simulink model "AAQuadModel"  (R2019b)
settings: Solver=VariableStepAuto  StartTime=0.0  StopTime=30.0  RelTol=1e-3
libraries: aerolibconvert2 x6, simulink x5, dspsigops x3, shared6dof x1, aerolibanim x1
settings Model: Creator=Antho  LastModifiedBy=Antho
settings SFSimCC: CustomCodeUndefinedFunction=UseInterfaceOnly

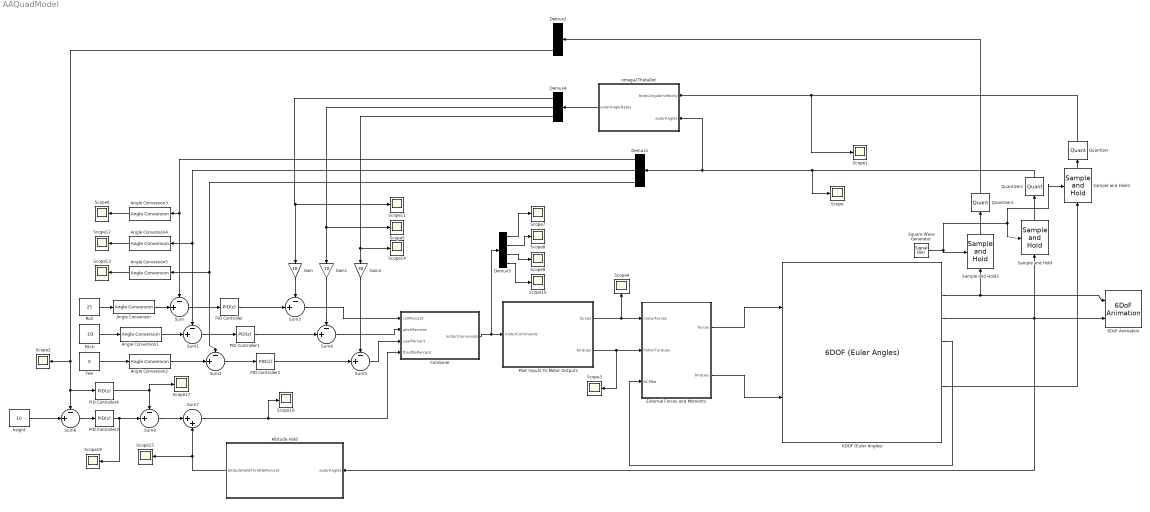
== system AAQuadModel ==
  6DOF (Euler Angles) : shared6dof/6DOF (Euler Angles)  units=Metric (MKS)  mtype=Fixed  rep=Euler Angles  xme_0=[0 0 0]  Vm_0=[0 0 0]  eul_0=[0 0 0]  pm_0=[0 0 0]  mass_0=0.5  mass_e=0.5  mass_f=2.0  inertia=[0.1 0 0; 0 0.1 0; 0 0 0.2]  inertia_e=eye(3)  inertia_f=2*eye(3)  k_quat=1.0  vre_flag=on  abi_flag=off  aMode=0  xme_statename=''  Vm_statename=''  eul_statename=''  quat_statename=''  pm_statename=''  mass_statename=''
      settings: SourceProductBaseCode=AE
  6DoF Animation : aerolibanim/6DoF Animation  u1=[0 4000 -2000 2000 -5000 -3000]  u2=0.1  u3=1.0  u4=[4000 0 -5000]  u5=Fixed position  u6=[2000 500 -3150]  u7=10  u8=on
      settings: SourceProductName=Aerospace Blockset
  Altitude Hold : MATLAB Function  TreatAsAtomicUnit=on
  Angle Conversion : aerolibconvert2/Angle Conversion  IU=deg  OU=rad
  Angle Conversion1 : aerolibconvert2/Angle Conversion  IU=deg  OU=rad
  Angle Conversion2 : aerolibconvert2/Angle Conversion  IU=deg  OU=rad
  Angle Conversion3 : aerolibconvert2/Angle Conversion  IU=rad  OU=deg
  Angle Conversion4 : aerolibconvert2/Angle Conversion  IU=rad  OU=deg
  Angle Conversion5 : aerolibconvert2/Angle Conversion  IU=rad  OU=deg
  "Combiner " : MATLAB Function  TreatAsAtomicUnit=on
  Demux1 : Demux  Outputs=3
  Demux2 : Demux  Outputs=3
  Demux3 : Demux
  Demux4 : Demux  Outputs=3
  "External Forces and Moments " : MATLAB Function  TreatAsAtomicUnit=on
  Gain : Gain  Gain=10
  Gain1 : Gain  Gain=10
  Gain2 : Gain  Gain=30
  PID Controller : simulink/Continuous/PID Controller  Controller=PID  Form=Parallel  TimeDomain=Discrete-time  SampleTime=0.02  IntegratorMethod=Forward Euler  FilterMethod=Forward Euler  ControllerParametersSource=internal  P=30  I=0.2  D=0  UseFilter=on  N=100  TunerSelectOption=Transfer Function Based (PID Tuner App)  InitialConditionSource=internal  InitialConditionForIntegrator=0  InitialConditionForFilter=0  DifferentiatorICPrevScaledInput=0  ExternalReset=none  TrackingMode=off  Kt=1  LimitOutput=on  UpperSaturationLimit=20  LowerSaturationLimit=-20  LinearizeAsGain=on  AntiWindupMode=none  Kb=1  POutMin=[]  POutMax=[]  IOutMin=[]  IOutMax=[]  DOutMin=[]  DOutMax=[]  NOutMin=[]  NOutMax=[]  SumOutMin=[]  SumOutMax=[]  SaturationOutMin=[]  SaturationOutMax=[]  PParamMin=[]  PParamMax=[]  IParamMin=[]  IParamMax=[]  DParamMin=[]  DParamMax=[]  NParamMin=[]  NParamMax=[]  KbParamMin=[]  KbParamMax=[]  KtParamMin=[]  KtParamMax=[]  KbOutMin=[]  KbOutMax=[]  KtOutMin=[]  KtOutMax=[]  IntegratorOutMin=[]  IntegratorOutMax=[]  FilterOutMin=[]  FilterOutMax=[]  SumI1OutMin=[]  SumI1OutMax=[]  SumI2OutMin=[]  SumI2OutMax=[]  SumI3OutMin=[]  SumI3OutMax=[]  SumI4OutMin=[]  SumI4OutMax=[]  SumDOutMin=[]  SumDOutMax=[]  DifferentiatorOutMin=[]  DifferentiatorOutMax=[]  FilterDiffOutCoefMin=[]  FilterDiffOutCoefMax=[]  ReciprocalOutMin=[]  ReciprocalOutMax=[]  SumDenOutMin=[]  SumDenOutMax=[]  SumNumOutMin=[]  SumNumOutMax=[]  DivideOutMin=[]  DivideOutMax=[]  IntegratorContinuousStateAttributes=''  IntegratorStateMustResolveToSignalObject=off  IntegratorRTWStateStorageClass=Auto  FilterContinuousStateAttributes=''  FilterStateMustResolveToSignalObject=off  FilterRTWStateStorageClass=Auto  ParallelPVariant=InternalParameters  IdealPVariant=Disabled  IVariant=InternalParameters  DVariant=InternalParameters  IntegratorVariant=Discrete  SatVariant=Enabled  AWVariant=Passthrough  PCopyVariant=Disabled  TRVariant=Disabled  FdbkBlocksVariant=Forward  IdealPFdbkVariant=Disabled  SatFdbkVariant=Disabled  DerivativeFilterVariant=ForwardEulerFilter  NVariant=InternalParameters  NCopyVariant=Disabled  FilterICVariant=InternalICsFilter  IntegratorICVariant=InternalICs  ExternalResetVariant=Disabled  TRSumVariant=Passthrough  SumFdbkVariant=Disabled  SumVariant=Sum_PID
  PID Controller1 : simulink/Continuous/PID Controller  Controller=PID  Form=Parallel  TimeDomain=Discrete-time  SampleTime=0.02  IntegratorMethod=Forward Euler  FilterMethod=Forward Euler  ControllerParametersSource=internal  P=30  I=0.2  D=0  UseFilter=on  N=100  TunerSelectOption=Transfer Function Based (PID Tuner App)  InitialConditionSource=internal  InitialConditionForIntegrator=0  InitialConditionForFilter=0  DifferentiatorICPrevScaledInput=0  ExternalReset=none  TrackingMode=off  Kt=1  LimitOutput=on  UpperSaturationLimit=20  LowerSaturationLimit=-20  LinearizeAsGain=on  AntiWindupMode=none  Kb=1  POutMin=[]  POutMax=[]  IOutMin=[]  IOutMax=[]  DOutMin=[]  DOutMax=[]  NOutMin=[]  NOutMax=[]  SumOutMin=[]  SumOutMax=[]  SaturationOutMin=[]  SaturationOutMax=[]  PParamMin=[]  PParamMax=[]  IParamMin=[]  IParamMax=[]  DParamMin=[]  DParamMax=[]  NParamMin=[]  NParamMax=[]  KbParamMin=[]  KbParamMax=[]  KtParamMin=[]  KtParamMax=[]  KbOutMin=[]  KbOutMax=[]  KtOutMin=[]  KtOutMax=[]  IntegratorOutMin=[]  IntegratorOutMax=[]  FilterOutMin=[]  FilterOutMax=[]  SumI1OutMin=[]  SumI1OutMax=[]  SumI2OutMin=[]  SumI2OutMax=[]  SumI3OutMin=[]  SumI3OutMax=[]  SumI4OutMin=[]  SumI4OutMax=[]  SumDOutMin=[]  SumDOutMax=[]  DifferentiatorOutMin=[]  DifferentiatorOutMax=[]  FilterDiffOutCoefMin=[]  FilterDiffOutCoefMax=[]  ReciprocalOutMin=[]  ReciprocalOutMax=[]  SumDenOutMin=[]  SumDenOutMax=[]  SumNumOutMin=[]  SumNumOutMax=[]  DivideOutMin=[]  DivideOutMax=[]  IntegratorContinuousStateAttributes=''  IntegratorStateMustResolveToSignalObject=off  IntegratorRTWStateStorageClass=Auto  FilterContinuousStateAttributes=''  FilterStateMustResolveToSignalObject=off  FilterRTWStateStorageClass=Auto  ParallelPVariant=InternalParameters  IdealPVariant=Disabled  IVariant=InternalParameters  DVariant=InternalParameters  IntegratorVariant=Discrete  SatVariant=Enabled  AWVariant=Passthrough  PCopyVariant=Disabled  TRVariant=Disabled  FdbkBlocksVariant=Forward  IdealPFdbkVariant=Disabled  SatFdbkVariant=Disabled  DerivativeFilterVariant=ForwardEulerFilter  NVariant=InternalParameters  NCopyVariant=Disabled  FilterICVariant=InternalICsFilter  IntegratorICVariant=InternalICs  ExternalResetVariant=Disabled  TRSumVariant=Passthrough  SumFdbkVariant=Disabled  SumVariant=Sum_PID
  PID Controller2 : simulink/Continuous/PID Controller  Controller=PID  Form=Parallel  TimeDomain=Discrete-time  SampleTime=0.02  IntegratorMethod=Forward Euler  FilterMethod=Forward Euler  ControllerParametersSource=internal  P=20  I=0.2  D=0  UseFilter=on  N=100  TunerSelectOption=Transfer Function Based (PID Tuner App)  InitialConditionSource=internal  InitialConditionForIntegrator=0  InitialConditionForFilter=0  DifferentiatorICPrevScaledInput=0  ExternalReset=none  TrackingMode=off  Kt=1  LimitOutput=on  UpperSaturationLimit=20  LowerSaturationLimit=-20  LinearizeAsGain=on  AntiWindupMode=none  Kb=1  POutMin=[]  POutMax=[]  IOutMin=[]  IOutMax=[]  DOutMin=[]  DOutMax=[]  NOutMin=[]  NOutMax=[]  SumOutMin=[]  SumOutMax=[]  SaturationOutMin=[]  SaturationOutMax=[]  PParamMin=[]  PParamMax=[]  IParamMin=[]  IParamMax=[]  DParamMin=[]  DParamMax=[]  NParamMin=[]  NParamMax=[]  KbParamMin=[]  KbParamMax=[]  KtParamMin=[]  KtParamMax=[]  KbOutMin=[]  KbOutMax=[]  KtOutMin=[]  KtOutMax=[]  IntegratorOutMin=[]  IntegratorOutMax=[]  FilterOutMin=[]  FilterOutMax=[]  SumI1OutMin=[]  SumI1OutMax=[]  SumI2OutMin=[]  SumI2OutMax=[]  SumI3OutMin=[]  SumI3OutMax=[]  SumI4OutMin=[]  SumI4OutMax=[]  SumDOutMin=[]  SumDOutMax=[]  DifferentiatorOutMin=[]  DifferentiatorOutMax=[]  FilterDiffOutCoefMin=[]  FilterDiffOutCoefMax=[]  ReciprocalOutMin=[]  ReciprocalOutMax=[]  SumDenOutMin=[]  SumDenOutMax=[]  SumNumOutMin=[]  SumNumOutMax=[]  DivideOutMin=[]  DivideOutMax=[]  IntegratorContinuousStateAttributes=''  IntegratorStateMustResolveToSignalObject=off  IntegratorRTWStateStorageClass=Auto  FilterContinuousStateAttributes=''  FilterStateMustResolveToSignalObject=off  FilterRTWStateStorageClass=Auto  ParallelPVariant=InternalParameters  IdealPVariant=Disabled  IVariant=InternalParameters  DVariant=InternalParameters  IntegratorVariant=Discrete  SatVariant=Enabled  AWVariant=Passthrough  PCopyVariant=Disabled  TRVariant=Disabled  FdbkBlocksVariant=Forward  IdealPFdbkVariant=Disabled  SatFdbkVariant=Disabled  DerivativeFilterVariant=ForwardEulerFilter  NVariant=InternalParameters  NCopyVariant=Disabled  FilterICVariant=InternalICsFilter  IntegratorICVariant=InternalICs  ExternalResetVariant=Disabled  TRSumVariant=Passthrough  SumFdbkVariant=Disabled  SumVariant=Sum_PID
  PID Controller3 : simulink/Continuous/PID Controller  Controller=PID  Form=Parallel  TimeDomain=Discrete-time  SampleTime=0.02  IntegratorMethod=Forward Euler  FilterMethod=Forward Euler  ControllerParametersSource=internal  P=3  I=1  D=0  UseFilter=on  N=100  TunerSelectOption=Transfer Function Based (PID Tuner App)  InitialConditionSource=internal  InitialConditionForIntegrator=0  InitialConditionForFilter=0  DifferentiatorICPrevScaledInput=0  ExternalReset=none  TrackingMode=off  Kt=1  LimitOutput=on  UpperSaturationLimit=20  LowerSaturationLimit=-20  LinearizeAsGain=on  AntiWindupMode=none  Kb=1  POutMin=[]  POutMax=[]  IOutMin=[]  IOutMax=[]  DOutMin=[]  DOutMax=[]  NOutMin=[]  NOutMax=[]  SumOutMin=[]  SumOutMax=[]  SaturationOutMin=[]  SaturationOutMax=[]  PParamMin=[]  PParamMax=[]  IParamMin=[]  IParamMax=[]  DParamMin=[]  DParamMax=[]  NParamMin=[]  NParamMax=[]  KbParamMin=[]  KbParamMax=[]  KtParamMin=[]  KtParamMax=[]  KbOutMin=[]  KbOutMax=[]  KtOutMin=[]  KtOutMax=[]  IntegratorOutMin=[]  IntegratorOutMax=[]  FilterOutMin=[]  FilterOutMax=[]  SumI1OutMin=[]  SumI1OutMax=[]  SumI2OutMin=[]  SumI2OutMax=[]  SumI3OutMin=[]  SumI3OutMax=[]  SumI4OutMin=[]  SumI4OutMax=[]  SumDOutMin=[]  SumDOutMax=[]  DifferentiatorOutMin=[]  DifferentiatorOutMax=[]  FilterDiffOutCoefMin=[]  FilterDiffOutCoefMax=[]  ReciprocalOutMin=[]  ReciprocalOutMax=[]  SumDenOutMin=[]  SumDenOutMax=[]  SumNumOutMin=[]  SumNumOutMax=[]  DivideOutMin=[]  DivideOutMax=[]  IntegratorContinuousStateAttributes=''  IntegratorStateMustResolveToSignalObject=off  IntegratorRTWStateStorageClass=Auto  FilterContinuousStateAttributes=''  FilterStateMustResolveToSignalObject=off  FilterRTWStateStorageClass=Auto  ParallelPVariant=InternalParameters  IdealPVariant=Disabled  IVariant=InternalParameters  DVariant=InternalParameters  IntegratorVariant=Discrete  SatVariant=Enabled  AWVariant=Passthrough  PCopyVariant=Disabled  TRVariant=Disabled  FdbkBlocksVariant=Forward  IdealPFdbkVariant=Disabled  SatFdbkVariant=Disabled  DerivativeFilterVariant=ForwardEulerFilter  NVariant=InternalParameters  NCopyVariant=Disabled  FilterICVariant=InternalICsFilter  IntegratorICVariant=InternalICs  ExternalResetVariant=Disabled  TRSumVariant=Passthrough  SumFdbkVariant=Disabled  SumVariant=Sum_PID
  PID Controller4 : simulink/Continuous/PID Controller  Controller=PID  Form=Parallel  TimeDomain=Discrete-time  SampleTime=0.02  IntegratorMethod=Forward Euler  FilterMethod=Forward Euler  ControllerParametersSource=internal  P=0  I=0  D=3  UseFilter=on  N=100  TunerSelectOption=Transfer Function Based (PID Tuner App)  InitialConditionSource=internal  InitialConditionForIntegrator=0  InitialConditionForFilter=0  DifferentiatorICPrevScaledInput=0  ExternalReset=none  TrackingMode=off  Kt=1  LimitOutput=on  UpperSaturationLimit=20  LowerSaturationLimit=-20  LinearizeAsGain=on  AntiWindupMode=none  Kb=1  POutMin=[]  POutMax=[]  IOutMin=[]  IOutMax=[]  DOutMin=[]  DOutMax=[]  NOutMin=[]  NOutMax=[]  SumOutMin=[]  SumOutMax=[]  SaturationOutMin=[]  SaturationOutMax=[]  PParamMin=[]  PParamMax=[]  IParamMin=[]  IParamMax=[]  DParamMin=[]  DParamMax=[]  NParamMin=[]  NParamMax=[]  KbParamMin=[]  KbParamMax=[]  KtParamMin=[]  KtParamMax=[]  KbOutMin=[]  KbOutMax=[]  KtOutMin=[]  KtOutMax=[]  IntegratorOutMin=[]  IntegratorOutMax=[]  FilterOutMin=[]  FilterOutMax=[]  SumI1OutMin=[]  SumI1OutMax=[]  SumI2OutMin=[]  SumI2OutMax=[]  SumI3OutMin=[]  SumI3OutMax=[]  SumI4OutMin=[]  SumI4OutMax=[]  SumDOutMin=[]  SumDOutMax=[]  DifferentiatorOutMin=[]  DifferentiatorOutMax=[]  FilterDiffOutCoefMin=[]  FilterDiffOutCoefMax=[]  ReciprocalOutMin=[]  ReciprocalOutMax=[]  SumDenOutMin=[]  SumDenOutMax=[]  SumNumOutMin=[]  SumNumOutMax=[]  DivideOutMin=[]  DivideOutMax=[]  IntegratorContinuousStateAttributes=''  IntegratorStateMustResolveToSignalObject=off  IntegratorRTWStateStorageClass=Auto  FilterContinuousStateAttributes=''  FilterStateMustResolveToSignalObject=off  FilterRTWStateStorageClass=Auto  ParallelPVariant=InternalParameters  IdealPVariant=Disabled  IVariant=InternalParameters  DVariant=InternalParameters  IntegratorVariant=Discrete  SatVariant=Enabled  AWVariant=Passthrough  PCopyVariant=Disabled  TRVariant=Disabled  FdbkBlocksVariant=Forward  IdealPFdbkVariant=Disabled  SatFdbkVariant=Disabled  DerivativeFilterVariant=ForwardEulerFilter  NVariant=InternalParameters  NCopyVariant=Disabled  FilterICVariant=InternalICsFilter  IntegratorICVariant=InternalICs  ExternalResetVariant=Disabled  TRSumVariant=Passthrough  SumFdbkVariant=Disabled  SumVariant=Sum_PID
  Pilot Inputs To Motor Outputs : MATLAB Function  TreatAsAtomicUnit=on
  Pitch : Constant  Value=-10
  Quantizer : Quantizer  QuantizationInterval=0.00003  LinearizeAsGain=off
  Quantizer1 : Quantizer  QuantizationInterval=0.00003  LinearizeAsGain=off
  Quantizer2 : Quantizer  QuantizationInterval=0.00003  LinearizeAsGain=off
  Roll : Constant  Value=25
  Sample and Hold : dspsigops/Sample and Hold  trig=Rising edge  initCond=0  latchinput=on
  Sample and Hold1 : dspsigops/Sample and Hold  trig=Rising edge  initCond=0  latchinput=on
  Sample and Hold2 : dspsigops/Sample and Hold  trig=Rising edge  initCond=0  latchinput=on
  Scope{,1..18} (19 alike) : Scope
  Square Wave Generator : SignalGenerator  WaveForm=square  Frequency=50
  Sum{,1..6,8} (8 alike) : Sum  Inputs=-+|
  Sum7 : Sum  Inputs=|++
  Yaw : Constant  Value=0
  height : Constant  Value=10
  omega2ThetaDot : MATLAB Function  TreatAsAtomicUnit=on
  wires:
  Pilot Inputs To Motor Outputs/1(forces) -> "External Forces and Moments "/1(motorForces), Scope4/1
  Pilot Inputs To Motor Outputs/2(torques) -> Scope3/1, "External Forces and Moments "/2(motorTorques)
  "External Forces and Moments "/1(forces) -> 6DOF (Euler Angles)/1
  "External Forces and Moments "/2(torques) -> 6DOF (Euler Angles)/2
  6DOF (Euler Angles)/4 -> "External Forces and Moments "/3(DCMbe)
  "Combiner "/1(motorCommands) -> Demux3/1, Pilot Inputs To Motor Outputs/1(motorCommands)
  Demux1/1 -> Angle Conversion3/1, Sum/1
  Sum/1 -> PID Controller/1
  Demux3/1 -> Scope7/1
  Demux3/2 -> Scope8/1
  Demux3/3 -> Scope9/1
  Demux3/4 -> Scope10/1
  6DOF (Euler Angles)/2 -> Sample and Hold2/1, 6DoF Animation/1
  Sum1/1 -> PID Controller1/1
  Demux1/2 -> Angle Conversion4/1, Sum1/1
  Sum2/1 -> PID Controller2/1
  Demux1/3 -> Angle Conversion5/1, Sum2/1
  PID Controller1/1 -> Sum4/2
  PID Controller/1 -> Sum3/2
  PID Controller2/1 -> Sum5/2
  omega2ThetaDot/1(eulerAngleRates) -> Demux4/1
  Gain1/1 -> Sum4/1
  Gain/1 -> Sum3/1
  Gain2/1 -> Sum5/1
  Sum5/1 -> "Combiner "/3(yawPercent)
  Sum4/1 -> "Combiner "/2(pitchPercent)
  Sum3/1 -> "Combiner "/1(rollPercent)
  Demux4/3 -> Scope14/1, Gain2/1
  Demux4/2 -> Scope5/1, Gain1/1
  Demux4/1 -> Scope11/1, Gain/1
  6DOF (Euler Angles)/6 -> Sample and Hold1/1
  Sample and Hold/1 -> Quantizer1/1
  Quantizer1/1 -> omega2ThetaDot/2(eulerAngles), Demux1/1, Scope/1
  Quantizer/1 -> Scope1/1, omega2ThetaDot/1(bodyAngularVelocity)
  Sample and Hold1/1 -> Quantizer/1
  Sample and Hold2/1 -> Quantizer2/1
  Square Wave Generator/1 -> Sample and Hold/Trigger, Sample and Hold1/Trigger, Sample and Hold2/Trigger
  Quantizer2/1 -> Demux2/1
  Demux2/3 -> Scope2/1, PID Controller4/1, Sum6/1
  height/1 -> Sum6/2
  Sum6/1 -> PID Controller3/1
  Sum7/1 -> "Combiner "/4(throttlePercent), Scope16/1
  Altitude Hold/1(altitudeHoldThrottlePercent) -> Scope15/1, Sum7/2
  6DOF (Euler Angles)/3 -> 6DoF Animation/2, Altitude Hold/1(eulerAngles), Sample and Hold/1
  Sum8/1 -> Sum7/1
  PID Controller3/1 -> Scope18/1, Sum8/2
  PID Controller4/1 -> Scope17/1, Sum8/1
  Angle Conversion/1 -> Sum/2
  Roll/1 -> Angle Conversion/1
  Angle Conversion1/1 -> Sum1/2
  Pitch/1 -> Angle Conversion1/1
  Angle Conversion2/1 -> Sum2/2
  Yaw/1 -> Angle Conversion2/1
  Angle Conversion5/1 -> Scope13/1
  Angle Conversion4/1 -> Scope12/1
  Angle Conversion3/1 -> Scope6/1

== matlab function AAQuadModel/External Forces and Moments  ==
  data: motorForces input; forces output; motorTorques input; DCMbe input; torques output
function [forces, torques] = fcn(motorForces, motorTorques, DCMbe)

mass = 0.5; % this is not real. Im using this nmber in the 6 dof block aswell.
gravityInertial = [0;0;-9.8*mass];
gravityBody = DCMbe.' * gravityInertial;

forces = motorForces + gravityBody;

torques = motorTorques;

== matlab function AAQuadModel/Pilot Inputs To Motor Outputs ==
  data: motorCommands input; forces output; torques output
function [forces, torques]= fcn(motorCommands)

forces = [0;0;0];
torques = [0;0;0];

% These values were calculated for the old quad model. 
% They will need to be experimentally recalculated with the new
% propeller/motor/battery combination.
percentToThrustFactor = 0.053508;
percentToThrustYIntercept = 0.7693;
thrustToTorqueFactorXY = 0.11;
thrustToTorqueFactorZ = 0.01;

forceOfMotor = [0;0;0;0];

for i=1:4
    if ((motorCommands(i) > 17) && (motorCommands(i) < 82)) % it was observed that below 17%, motors did not turn at all and over 82%, they did not accelerate
        forceOfMotor(i) = forces(3) + motorCommands(i)*percentToThrustFactor - percentToThrustYIntercept;
    elseif (motorCommands(i) >= 82)
        motorCommands(i) = 82;
        forceOfMotor(i) = forces(3) + motorCommands(i)*percentToThrustFactor - percentToThrustYIntercept;
    elseif (motorCommands(i) <= 17)
        motorCommands(i) = 17;
        forceOfMotor(i) = forces(3) + motorCommands(i)*percentToThrustFactor - percentToThrustYIntercept;
    end
end

forces(3) = sum(forceOfMotor);
torques(1) = ((forceOfMotor(1) + forceOfMotor(4)) - (forceOfMotor(2) +forceOfMotor(3))) * thrustToTorqueFactorXY;
torques(2) = ((forceOfMotor(1) + forceOfMotor(2)) - (forceOfMotor(3) +forceOfMotor(4))) * thrustToTorqueFactorXY; 
torques(3) = ((forceOfMotor(1) + forceOfMotor(3)) - (forceOfMotor(2) +forceOfMotor(4))) * thrustToTorqueFactorZ;

== matlab function AAQuadModel/Combiner  ==
  data: rollPercent input; motorCommands output; pitchPercent input; yawPercent input; throttlePercent input
function motorCommands = fcn(rollPercent, pitchPercent, yawPercent, throttlePercent)

motorCommands = [0;0;0;0];

motorCommands(1) = throttlePercent + rollPercent + pitchPercent + yawPercent;
motorCommands(2) = throttlePercent - rollPercent + pitchPercent - yawPercent;
motorCommands(3) = throttlePercent - rollPercent - pitchPercent + yawPercent;
motorCommands(4) = throttlePercent + rollPercent - pitchPercent - yawPercent;

== matlab function AAQuadModel/omega2ThetaDot ==
  data: bodyAngularVelocity input; eulerAngleRates output; eulerAngles input
function eulerAngleRates = fcn(bodyAngularVelocity, eulerAngles)

% The math showed phi was not relevant in computing the matrix
theta = eulerAngles(2);
psi = eulerAngles(3);

omega2ThetaDotMatrix=[
                        cos(psi)/cos(theta)  -sin(psi)/cos(theta) 0;
                        sin(psi)             cos(psi)             0;
                        -tan(theta)*cos(psi) tan(theta)*sin(psi)  1;
                     ]
eulerAngleRates = omega2ThetaDotMatrix*bodyAngularVelocity;

== matlab function AAQuadModel/Altitude Hold ==
  data: eulerAngles input; altitudeHoldThrottlePercent output
function altitudeHoldThrottlePercent = fcn(eulerAngles)

%todo the number 37 will need to be recalculated once the weight and thrust
%curve of the quad are known.
motorPercentLevelAltitudeHold = 37;

phi = eulerAngles(1);
theta = eulerAngles(2);


altitudeHoldThrottlePercent = motorPercentLevelAltitudeHold/(cos(phi)*cos(theta));
